simulink model "CTmodel"  (R2017a)
settings: Solver=VariableStepAuto  StartTime=0.0  StopTime=Ts  FixedStep=0.001  RelTol=1e-3
undefined symbols (not defined in the file or in its folder): magnitude, umpc, x
settings Model: Creator=s144470  LastModifiedBy=s144470

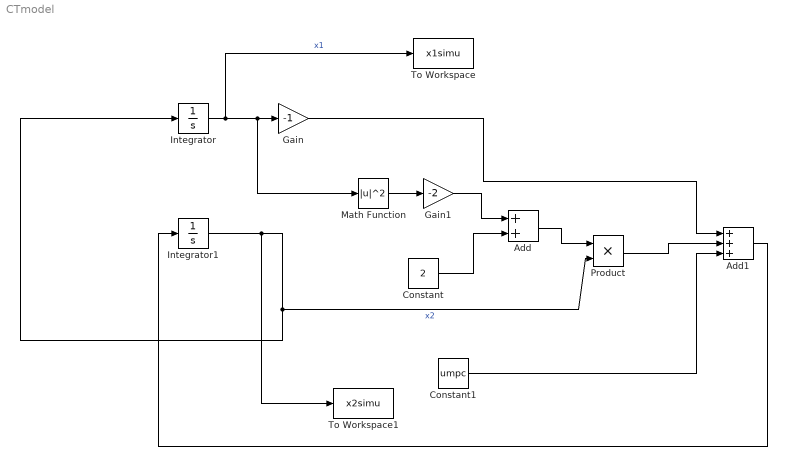
== system CTmodel ==
  Add : Sum
  Add1 : Sum  Inputs=+++
  Constant : Constant  Value=2
  Constant1 : Constant  Value=umpc
  Gain : Gain  Gain=-1
  Gain1 : Gain  Gain=-2
  Integrator : Integrator  InitialCondition=x(1)
  Integrator1 : Integrator  InitialCondition=x(2)
  Math Function : Math  Operator=magnitude^2  SaturateOnIntegerOverflow=on
  Product : Product
  To Workspace : ToWorkspace  VariableName=x1simu  SampleTime=-1
  To Workspace1 : ToWorkspace  VariableName=x2simu  SampleTime=-1
  wires:
  Integrator/1 -> To Workspace/1, Math Function/1, Gain/1  "x1"
  Integrator1/1 -> To Workspace1/1, Product/2, Integrator/1  "x2"
  Math Function/1 -> Gain1/1
  Constant/1 -> Add/2
  Gain1/1 -> Add/1
  Add/1 -> Product/1
  Gain/1 -> Add1/1
  Product/1 -> Add1/2
  Constant1/1 -> Add1/3
  Add1/1 -> Integrator1/1
